simulink model "com_process"  (R2021a)
settings: configuration reference "f2_ctrl_config" (kept outside this file)
settings Model: DataDictionary=motor_data.sldd  Creator=Litao  LastModifiedBy=Litao
settings ConfigSetRef: SourceName=f2_ctrl_config

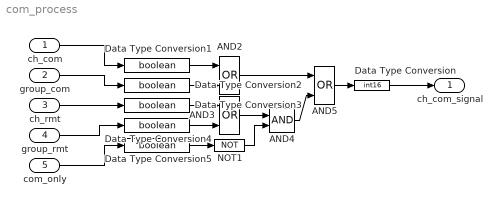
== system com_process ==
  ch_com : Inport  OutDataTypeStr=int16
  group_com : Inport  Port=2  OutDataTypeStr=int16
  ch_rmt : Inport  Port=3  OutDataTypeStr=int16
  group_rmt : Inport  Port=4  OutDataTypeStr=int16
  com_only : Inport  Port=5  OutDataTypeStr=int16
  AND2 : Logic  Operator=OR  AllPortsSameDT=off  OutDataTypeStr=boolean
  AND3 : Logic  Operator=OR  AllPortsSameDT=off  OutDataTypeStr=boolean
  AND4 : Logic  AllPortsSameDT=off  OutDataTypeStr=boolean
  AND5 : Logic  Operator=OR  AllPortsSameDT=off  OutDataTypeStr=boolean
  Data Type Conversion : DataTypeConversion  OutDataTypeStr=int16
  Data Type Conversion{1..5} (5 alike) : DataTypeConversion  OutDataTypeStr=boolean
  NOT1 : Logic  Operator=NOT  AllPortsSameDT=off  OutDataTypeStr=boolean
  ch_com_signal : Outport  OutDataTypeStr=int16
  wires:
  NOT1/1 -> AND4/2
  Data Type Conversion1/1 -> AND2/1
  Data Type Conversion3/1 -> AND3/1
  AND3/1 -> AND4/1
  AND2/1 -> AND5/1
  Data Type Conversion2/1 -> AND2/2
  AND4/1 -> AND5/2
  Data Type Conversion5/1 -> NOT1/1
  Data Type Conversion4/1 -> AND3/2
  AND5/1 -> Data Type Conversion/1
  ch_com/1 -> Data Type Conversion1/1
  group_com/1 -> Data Type Conversion2/1
  ch_rmt/1 -> Data Type Conversion3/1
  group_rmt/1 -> Data Type Conversion4/1
  com_only/1 -> Data Type Conversion5/1
  Data Type Conversion/1 -> ch_com_signal/1
